simulink model "RoboBoatVU_2014_Bacchus"  (R2014a)
settings: Solver=FixedStepDiscrete  StartTime=0.0  StopTime=inf  FixedStep=.1  RelTol=1e-3
undefined symbols (not defined in the file): Com1, Com2, Com3, Com4, DiscIntNeverNeededParam, RGB24, standard
libraries: visiontextngfix x51, simulink x44, xpcseriallib x15, dspmtrx3 x14, speedgoatlib_IO102 x3, slrtlib x2, visionstatistics x2, dspstat3 x2, dspindex x2, xpcvideousblib x2, xpcvideoutillib x2, speedgoatlib x1
(part 4 of 5)

== system RoboBoatVU_2014_Bacchus/Main FSM/Start Speed Gate/Buoy Decisions/Annotate Image ==
  RGB image : Inport
  Red BBox : Inport  Port=2
  Green BBox : Inport  Port=3
  Red Dist : Inport  Port=4
  Green Dist : Inport  Port=5
  Annotate Task : visiontextngfix/Insert Text  inputType=Obsolete  theText='Buoy Navigation'  getTextLocFrom=Specify via dialog  textLoc=[10 10]  getTextColorFrom=Specify via dialog  textColor=[0 0 255]  getTextIntensityFrom=Specify via dialog  textIntensity=0  getTextOpacityFrom=Specify via dialog  textOpacity=1.0  dummyVar2=0  dummyVar3=0  dummyVar4=0  imagePorts=One multidimensional signal  isInputTransposed=off  fontFace=LucidaSansRegular  dummyVar1=0  blockFontSize=12  antiAliased=on
  Draw Green BBox : visiontextngfix/Draw Shapes  shape=Rectangles  fill=on  lineWidth=1  fillClrSource=Specify via dialog  display=User-specified value  intensity=200  color=[0 255 0]  opacity=0.6  viewport=Entire image  antialiasing=off  inType=Obsolete  imagePorts=One multidimensional signal  prodOutputMode=Binary point scaling  prodOutputWordLength=32  prodOutputFracLength=14  memoryMode=Specify word length  memoryWordLength=16  memoryFracLength=14  roundingMode=Floor  overflowMode=off
  Draw Red BBox : visiontextngfix/Draw Shapes  shape=Rectangles  fill=on  lineWidth=1  fillClrSource=Specify via dialog  display=User-specified value  intensity=200  color=[255 0 0]  opacity=0.6  viewport=Entire image  antialiasing=off  inType=Obsolete  imagePorts=One multidimensional signal  prodOutputMode=Binary point scaling  prodOutputWordLength=32  prodOutputFracLength=14  memoryMode=Specify word length  memoryWordLength=16  memoryFracLength=14  roundingMode=Floor  overflowMode=off
  Green Distance Display : visiontextngfix/Insert Text  inputType=Obsolete  theText='Green Distance: %f m'  getTextLocFrom=Specify via dialog  textLoc=[10 130]  getTextColorFrom=Specify via dialog  textColor=[0 255 0]  getTextIntensityFrom=Specify via dialog  textIntensity=0  getTextOpacityFrom=Specify via dialog  textOpacity=1.0  dummyVar2=0  dummyVar3=0  dummyVar4=0  imagePorts=One multidimensional signal  isInputTransposed=off  fontFace=LucidaSansRegular  dummyVar1=0  blockFontSize=12  antiAliased=on
  Green integer : DataTypeConversion  OutDataTypeStr=int32
  Red Distance Display : visiontextngfix/Insert Text  inputType=Obsolete  theText='Red Distance: %f m'  getTextLocFrom=Specify via dialog  textLoc=[10 70]  getTextColorFrom=Specify via dialog  textColor=[255 0 0]  getTextIntensityFrom=Specify via dialog  textIntensity=0  getTextOpacityFrom=Specify via dialog  textOpacity=1.0  dummyVar2=0  dummyVar3=0  dummyVar4=0  imagePorts=One multidimensional signal  isInputTransposed=off  fontFace=LucidaSansRegular  dummyVar1=0  blockFontSize=12  antiAliased=on
  Red integer : DataTypeConversion  OutDataTypeStr=int32
  Annotated Image : Outport
  wires:
  RGB image/1 -> Draw Red BBox/1
  Red BBox/1 -> Red integer/1
  Red integer/1 -> Draw Red BBox/2
  Draw Red BBox/1 -> Draw Green BBox/1
  Green BBox/1 -> Green integer/1
  Draw Green BBox/1 -> Annotate Task/1
  Annotate Task/1 -> Red Distance Display/1
  Red Dist/1 -> Red Distance Display/2
  Green Distance Display/1 -> Annotated Image/1
  Red Distance Display/1 -> Green Distance Display/1
  Green Dist/1 -> Green Distance Display/2
  Green integer/1 -> Draw Green BBox/2

== system RoboBoatVU_2014_Bacchus/Main FSM/Start Speed Gate/Start Speed Gate Detection/Green Detection ==
  HSV : Inport
  Blob Analysis : visionstatistics/Blob Analysis  Tag=vipblks_row_conv  area=on  centroid=on  bBox=on  majorAxis=off  minorAxis=off  angle=off  eccentricity=off  equivDiameterSq=off  extent=on  perimeter=off  maxBlobs=4  warnIfNumBlobsExceeded=on  isCount=off  useMinArea=on  minArea=130  useMaxArea=off  maxArea=6000  excludeBorderBlob=off  outDT=double  isOutVarDim=off  isFill=on  fillValues=-1  conn=8  isLabel=off  outputMode=Binary point scaling  outputWordLength=32  outputFracLength=16  firstCoeffMode=Binary point scaling  firstCoeffWordLength=16  firstCoeffFracLength=14  secondCoeffMode=Binary point scaling  secondCoeffWordLength=32  secondCoeffFracLength=16  accumMode=Binary point scaling  accumWordLength=32  accumFracLength=0  prodOutputMode=Binary point scaling  prodOutputWordLength=32  prodOutputFracLength=16  roundingMode=Floor  overflowMode=off
  Exclusions1 : Subsystem
  Image Reduction : Subsystem
  y-shift : MATLAB Function  Commented=through  TreatAsAtomicUnit=on
  Green Centroid : Outport
  Green BBox : Outport  Port=2
  wires:
  HSV/1 -> Image Reduction/1(HSV)
  Exclusions1/1(Centroid Out) -> y-shift/1(CentroidIn)
  Exclusions1/2(BBox Out) -> y-shift/2(BBoxIn)
  y-shift/1(CentroidOut) -> Green Centroid/1
  y-shift/2(BBoxOut) -> Green BBox/1
  Blob Analysis/2 -> Exclusions1/2(Centroid In)
  Blob Analysis/1 -> Exclusions1/1(Area In)
  Blob Analysis/3 -> Exclusions1/3(BBox In)
  Blob Analysis/4 -> Exclusions1/4(Extent In)
  Image Reduction/1(Green BW) -> Blob Analysis/1

== system RoboBoatVU_2014_Bacchus/Main FSM/Start Speed Gate/Start Speed Gate Detection/Red Detection ==
  HSV : Inport
  Blob Analysis : visionstatistics/Blob Analysis  Tag=vipblks_row_conv  area=on  centroid=on  bBox=on  majorAxis=off  minorAxis=off  angle=off  eccentricity=off  equivDiameterSq=off  extent=on  perimeter=off  maxBlobs=4  warnIfNumBlobsExceeded=on  isCount=off  useMinArea=on  minArea=130  useMaxArea=off  maxArea=6000  excludeBorderBlob=off  outDT=double  isOutVarDim=off  isFill=on  fillValues=-1  conn=8  isLabel=off  outputMode=Binary point scaling  outputWordLength=32  outputFracLength=16  firstCoeffMode=Binary point scaling  firstCoeffWordLength=16  firstCoeffFracLength=14  secondCoeffMode=Binary point scaling  secondCoeffWordLength=32  secondCoeffFracLength=16  accumMode=Binary point scaling  accumWordLength=32  accumFracLength=0  prodOutputMode=Binary point scaling  prodOutputWordLength=32  prodOutputFracLength=16  roundingMode=Floor  overflowMode=off
  Exclusions : Subsystem
  Image Reduction : Subsystem
  y-shift : MATLAB Function  Commented=through  TreatAsAtomicUnit=on
  Red Centroid : Outport
  Red BBox : Outport  Port=2
  wires:
  HSV/1 -> Image Reduction/1(HSV)
  Exclusions/1(Centroid Out) -> y-shift/1(CentroidIn)
  Exclusions/2(BBox Out) -> y-shift/2(BBoxIn)
  y-shift/2(BBoxOut) -> Red BBox/1
  y-shift/1(CentroidOut) -> Red Centroid/1
  Blob Analysis/4 -> Exclusions/4(Extent In)
  Blob Analysis/2 -> Exclusions/2(Centroid In)
  Blob Analysis/1 -> Exclusions/1(Area In)
  Blob Analysis/3 -> Exclusions/3(BBox In)
  Image Reduction/1(Red BW) -> Blob Analysis/1

== system RoboBoatVU_2014_Bacchus/Sensors/Serial In/Decode Compass/Correct Heading Angle Magnetic to True North ==
  Heading Mag : Inport
  Magnetic Declination : Constant  Value=-10.877
  Magnetic to True North Conversion : MATLAB Function  TreatAsAtomicUnit=on
  Heading True : Outport
  wires:
  Magnetic to True North Conversion/1(HeadingT) -> Heading True/1  "Heading"
  Heading Mag/1 -> Magnetic to True North Conversion/1(HeadingM)
  Magnetic Declination/1 -> Magnetic to True North Conversion/2(MagDec)

== system RoboBoatVU_2014_Bacchus/Sinks/actuators/analog output/Subsystem ==
  Compass Heading : Inport
  Control Signals : Inport  Port=2
  Bus Selector : BusSelector  OutputSignals=RPM,Desired Heading
  Heading Controller : Subsystem
  Propulsion Controller : Subsystem
  Propulsion : Outport
  Steering : Outport  Port=2
  wires:
  Control Signals/1 -> Bus Selector/1
  Bus Selector/1 -> Propulsion Controller/1(RPM)  "<RPM>"
  Propulsion Controller/1(Propulsion) -> Propulsion/1
  Bus Selector/2 -> Heading Controller/1(Heading Desired)  "<Desired Heading>"
  Compass Heading/1 -> Heading Controller/2(Compass Heading)
  Heading Controller/1(Steering) -> Steering/1

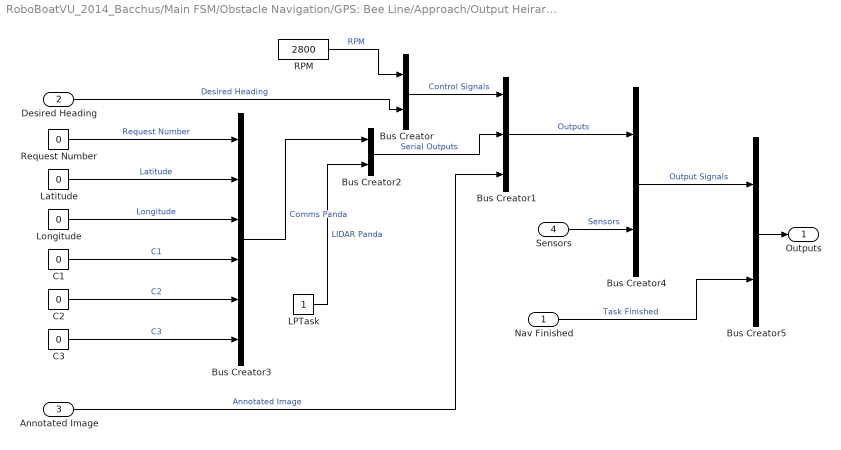
== system RoboBoatVU_2014_Bacchus/Main FSM/Obstacle Navigation/GPS: Bee Line/Approach/Output Heirarchy1 ==
  Nav Finished : Inport
  Desired Heading : Inport  Port=2
  Annotated Image : Inport  Port=3
  Sensors : Inport  Port=4
  Bus Creator{,2,4..5} (4 alike) : BusCreator  Inputs=2
  Bus Creator1 : BusCreator  Inputs=3
  Bus Creator3 : BusCreator  Inputs=6
  C1 : Constant  Value=0
  C2 : Constant  Value=0
  C3 : Constant  Value=0
  LPTask : Constant
  Latitude : Constant  Value=0
  Longitude : Constant  Value=0
  RPM : Constant  Value=2800
  Request Number : Constant  Value=0
  Outputs : Outport
  wires:
  RPM/1 -> Bus Creator/1  "RPM"
  Bus Creator/1 -> Bus Creator1/1  "Control Signals"
  Bus Creator3/1 -> Bus Creator2/1  "Comms Panda"
  Request Number/1 -> Bus Creator3/1  "Request Number"
  Latitude/1 -> Bus Creator3/2  "Latitude"
  Longitude/1 -> Bus Creator3/3  "Longitude"
  C1/1 -> Bus Creator3/4  "C1"
  LPTask/1 -> Bus Creator2/2  "LIDAR Panda"
  Desired Heading/1 -> Bus Creator/2  "Desired Heading"
  Bus Creator1/1 -> Bus Creator4/1  "Outputs"
  Annotated Image/1 -> Bus Creator1/3  "Annotated Image"
  Sensors/1 -> Bus Creator4/2  "Sensors"
  Bus Creator4/1 -> Bus Creator5/1  "Output Signals"
  Bus Creator2/1 -> Bus Creator1/2  "Serial Outputs"
  C2/1 -> Bus Creator3/5  "C2"
  C3/1 -> Bus Creator3/6  "C3"
  Nav Finished/1 -> Bus Creator5/2  "Task Finished"
  Bus Creator5/1 -> Outputs/1

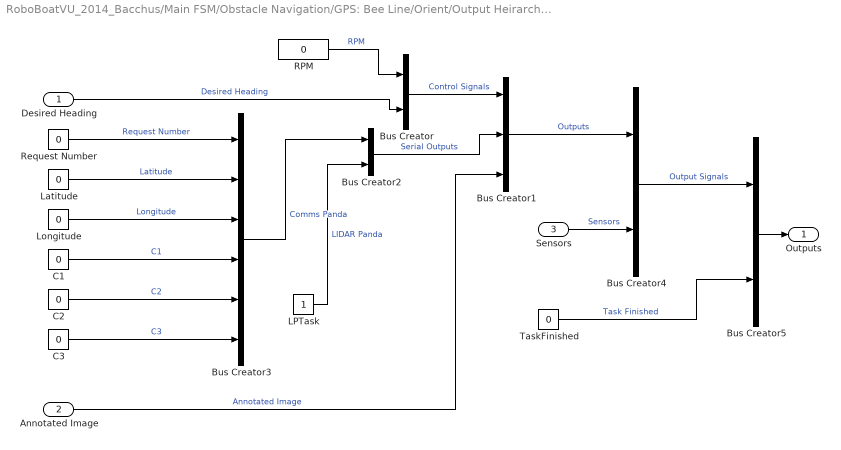
== system RoboBoatVU_2014_Bacchus/Main FSM/Obstacle Navigation/GPS: Bee Line/Orient/Output Heirarchy1 ==
  Desired Heading : Inport
  Annotated Image : Inport  Port=2
  Sensors : Inport  Port=3
  Bus Creator{,2,4..5} (4 alike) : BusCreator  Inputs=2
  Bus Creator1 : BusCreator  Inputs=3
  Bus Creator3 : BusCreator  Inputs=6
  C1 : Constant  Value=0
  C2 : Constant  Value=0
  C3 : Constant  Value=0
  LPTask : Constant
  Latitude : Constant  Value=0
  Longitude : Constant  Value=0
  RPM : Constant  Value=0
  Request Number : Constant  Value=0
  TaskFinished : Constant  Value=0
  Outputs : Outport
  wires:
  RPM/1 -> Bus Creator/1  "RPM"
  Bus Creator/1 -> Bus Creator1/1  "Control Signals"
  Bus Creator3/1 -> Bus Creator2/1  "Comms Panda"
  Request Number/1 -> Bus Creator3/1  "Request Number"
  Latitude/1 -> Bus Creator3/2  "Latitude"
  Longitude/1 -> Bus Creator3/3  "Longitude"
  C1/1 -> Bus Creator3/4  "C1"
  LPTask/1 -> Bus Creator2/2  "LIDAR Panda"
  Desired Heading/1 -> Bus Creator/2  "Desired Heading"
  Bus Creator1/1 -> Bus Creator4/1  "Outputs"
  Annotated Image/1 -> Bus Creator1/3  "Annotated Image"
  Sensors/1 -> Bus Creator4/2  "Sensors"
  Bus Creator4/1 -> Bus Creator5/1  "Output Signals"
  Bus Creator2/1 -> Bus Creator1/2  "Serial Outputs"
  C2/1 -> Bus Creator3/5  "C2"
  C3/1 -> Bus Creator3/6  "C3"
  TaskFinished/1 -> Bus Creator5/2  "Task Finished"
  Bus Creator5/1 -> Outputs/1

== system RoboBoatVU_2014_Bacchus/Main FSM/Obstacle Navigation1/Enter Gate/Gate 1 (Red & White)/Output Heirarchy ==
  Annotated Image : Inport
  Sensors : Inport  Port=2
  RPM : Inport  Port=3
  Desired Heading : Inport  Port=4
  Task Finished : Inport  Port=5
  Bus Creator : BusCreator  Inputs=3
  Bus Creator1 : BusCreator  Inputs=2
  Bus Creator2 : BusCreator  Inputs=3
  Bus Creator3 : BusCreator  Inputs=2
  Bus Creator4 : BusCreator  Inputs=2
  Due Sample Start : Constant  Value=0
  Ready to Read : Constant  Value=0
  Uno Power : Constant  Value=0
  Outputs : Outport
  wires:
  RPM/1 -> Bus Creator/1  "RPM"
  Bus Creator/1 -> Bus Creator1/1  "Control Signals"
  Bus Creator2/1 -> Bus Creator/3  "Arduino Signals"
  Uno Power/1 -> Bus Creator2/2  "Uno Power"
  Desired Heading/1 -> Bus Creator/2  "Desired Heading"
  Bus Creator1/1 -> Bus Creator4/1  "Outputs"
  Annotated Image/1 -> Bus Creator1/2  "Annotated Image"
  Sensors/1 -> Bus Creator4/2  "Sensors"
  Bus Creator4/1 -> Bus Creator3/1  "Output Signals"
  Ready to Read/1 -> Bus Creator2/1  "Ready to Read"
  Due Sample Start/1 -> Bus Creator2/3  "Due Sample Start"
  Task Finished/1 -> Bus Creator3/2  "Task Finished"
  Bus Creator3/1 -> Outputs/1

== system RoboBoatVU_2014_Bacchus/Main FSM/Obstacle Navigation1/Enter Gate/Gate 2 (White & White)/Output Heirarchy ==
  Annotated Image : Inport
  Sensors : Inport  Port=2
  RPM : Inport  Port=3
  Desired Heading : Inport  Port=4
  Task Finished : Inport  Port=5
  Bus Creator : BusCreator  Inputs=3
  Bus Creator1 : BusCreator  Inputs=2
  Bus Creator2 : BusCreator  Inputs=3
  Bus Creator3 : BusCreator  Inputs=2
  Bus Creator4 : BusCreator  Inputs=2
  Due Sample Start : Constant  Value=0
  Ready to Read : Constant  Value=0
  Uno Power : Constant  Value=0
  Outputs : Outport
  wires:
  RPM/1 -> Bus Creator/1  "RPM"
  Bus Creator/1 -> Bus Creator1/1  "Control Signals"
  Bus Creator2/1 -> Bus Creator/3  "Arduino Signals"
  Uno Power/1 -> Bus Creator2/2  "Uno Power"
  Desired Heading/1 -> Bus Creator/2  "Desired Heading"
  Bus Creator1/1 -> Bus Creator4/1  "Outputs"
  Annotated Image/1 -> Bus Creator1/2  "Annotated Image"
  Sensors/1 -> Bus Creator4/2  "Sensors"
  Bus Creator4/1 -> Bus Creator3/1  "Output Signals"
  Ready to Read/1 -> Bus Creator2/1  "Ready to Read"
  Due Sample Start/1 -> Bus Creator2/3  "Due Sample Start"
  Task Finished/1 -> Bus Creator3/2  "Task Finished"
  Bus Creator3/1 -> Outputs/1

== system RoboBoatVU_2014_Bacchus/Main FSM/Obstacle Navigation1/Enter Gate/Gate 3 (White & Green)/Output Heirarchy ==
  Annotated Image : Inport
  Sensors : Inport  Port=2
  RPM : Inport  Port=3
  Desired Heading : Inport  Port=4
  Task Finished : Inport  Port=5
  Bus Creator : BusCreator  Inputs=3
  Bus Creator1 : BusCreator  Inputs=2
  Bus Creator2 : BusCreator  Inputs=3
  Bus Creator3 : BusCreator  Inputs=2
  Bus Creator4 : BusCreator  Inputs=2
  Due Sample Start : Constant  Value=0
  Ready to Read : Constant  Value=0
  Uno Power : Constant  Value=0
  Outputs : Outport
  wires:
  RPM/1 -> Bus Creator/1  "RPM"
  Bus Creator/1 -> Bus Creator1/1  "Control Signals"
  Bus Creator2/1 -> Bus Creator/3  "Arduino Signals"
  Uno Power/1 -> Bus Creator2/2  "Uno Power"
  Desired Heading/1 -> Bus Creator/2  "Desired Heading"
  Bus Creator1/1 -> Bus Creator4/1  "Outputs"
  Annotated Image/1 -> Bus Creator1/2  "Annotated Image"
  Sensors/1 -> Bus Creator4/2  "Sensors"
  Bus Creator4/1 -> Bus Creator3/1  "Output Signals"
  Ready to Read/1 -> Bus Creator2/1  "Ready to Read"
  Due Sample Start/1 -> Bus Creator2/3  "Due Sample Start"
  Task Finished/1 -> Bus Creator3/2  "Task Finished"
  Bus Creator3/1 -> Outputs/1

== system RoboBoatVU_2014_Bacchus/Main FSM/Obstacle Navigation1/Exit Gate/Gate 1 (Red & White)/Output Heirarchy ==
  Annotated Image : Inport
  Sensors : Inport  Port=2
  RPM : Inport  Port=3
  Desired Heading : Inport  Port=4
  Task Finished : Inport  Port=5
  Bus Creator : BusCreator  Inputs=3
  Bus Creator1 : BusCreator  Inputs=2
  Bus Creator2 : BusCreator  Inputs=3
  Bus Creator3 : BusCreator  Inputs=2
  Bus Creator4 : BusCreator  Inputs=2
  Due Sample Start : Constant  Value=0
  Ready to Read : Constant  Value=0
  Uno Power : Constant  Value=0
  Outputs : Outport
  wires:
  RPM/1 -> Bus Creator/1  "RPM"
  Bus Creator/1 -> Bus Creator1/1  "Control Signals"
  Bus Creator2/1 -> Bus Creator/3  "Arduino Signals"
  Uno Power/1 -> Bus Creator2/2  "Uno Power"
  Desired Heading/1 -> Bus Creator/2  "Desired Heading"
  Bus Creator1/1 -> Bus Creator4/1  "Outputs"
  Annotated Image/1 -> Bus Creator1/2  "Annotated Image"
  Sensors/1 -> Bus Creator4/2  "Sensors"
  Bus Creator4/1 -> Bus Creator3/1  "Output Signals"
  Ready to Read/1 -> Bus Creator2/1  "Ready to Read"
  Due Sample Start/1 -> Bus Creator2/3  "Due Sample Start"
  Task Finished/1 -> Bus Creator3/2  "Task Finished"
  Bus Creator3/1 -> Outputs/1

== system RoboBoatVU_2014_Bacchus/Main FSM/Obstacle Navigation1/Exit Gate/Gate 2 (White & White)/Output Heirarchy ==
  Annotated Image : Inport
  Sensors : Inport  Port=2
  RPM : Inport  Port=3
  Desired Heading : Inport  Port=4
  Task Finished : Inport  Port=5
  Bus Creator : BusCreator  Inputs=3
  Bus Creator1 : BusCreator  Inputs=2
  Bus Creator2 : BusCreator  Inputs=3
  Bus Creator3 : BusCreator  Inputs=2
  Bus Creator4 : BusCreator  Inputs=2
  Due Sample Start : Constant  Value=0
  Ready to Read : Constant  Value=0
  Uno Power : Constant  Value=0
  Outputs : Outport
  wires:
  RPM/1 -> Bus Creator/1  "RPM"
  Bus Creator/1 -> Bus Creator1/1  "Control Signals"
  Bus Creator2/1 -> Bus Creator/3  "Arduino Signals"
  Uno Power/1 -> Bus Creator2/2  "Uno Power"
  Desired Heading/1 -> Bus Creator/2  "Desired Heading"
  Bus Creator1/1 -> Bus Creator4/1  "Outputs"
  Annotated Image/1 -> Bus Creator1/2  "Annotated Image"
  Sensors/1 -> Bus Creator4/2  "Sensors"
  Bus Creator4/1 -> Bus Creator3/1  "Output Signals"
  Ready to Read/1 -> Bus Creator2/1  "Ready to Read"
  Due Sample Start/1 -> Bus Creator2/3  "Due Sample Start"
  Task Finished/1 -> Bus Creator3/2  "Task Finished"
  Bus Creator3/1 -> Outputs/1

== system RoboBoatVU_2014_Bacchus/Main FSM/Obstacle Navigation1/Exit Gate/Gate 3 (White & Green)/Output Heirarchy ==
  Annotated Image : Inport
  Sensors : Inport  Port=2
  RPM : Inport  Port=3
  Desired Heading : Inport  Port=4
  Task Finished : Inport  Port=5
  Bus Creator : BusCreator  Inputs=3
  Bus Creator1 : BusCreator  Inputs=2
  Bus Creator2 : BusCreator  Inputs=3
  Bus Creator3 : BusCreator  Inputs=2
  Bus Creator4 : BusCreator  Inputs=2
  Due Sample Start : Constant  Value=0
  Ready to Read : Constant  Value=0
  Uno Power : Constant  Value=0
  Outputs : Outport
  wires:
  RPM/1 -> Bus Creator/1  "RPM"
  Bus Creator/1 -> Bus Creator1/1  "Control Signals"
  Bus Creator2/1 -> Bus Creator/3  "Arduino Signals"
  Uno Power/1 -> Bus Creator2/2  "Uno Power"
  Desired Heading/1 -> Bus Creator/2  "Desired Heading"
  Bus Creator1/1 -> Bus Creator4/1  "Outputs"
  Annotated Image/1 -> Bus Creator1/2  "Annotated Image"
  Sensors/1 -> Bus Creator4/2  "Sensors"
  Bus Creator4/1 -> Bus Creator3/1  "Output Signals"
  Ready to Read/1 -> Bus Creator2/1  "Ready to Read"
  Due Sample Start/1 -> Bus Creator2/3  "Due Sample Start"
  Task Finished/1 -> Bus Creator3/2  "Task Finished"
  Bus Creator3/1 -> Outputs/1

== system RoboBoatVU_2014_Bacchus/Main FSM/Obstacle Navigation1/GPS: Center/Approach/Output Heirarchy ==
  Finished : Inport
  Desired Heading : Inport  Port=2
  Annotated Image : Inport  Port=3
  Sensors : Inport  Port=4
  Bus Creator : BusCreator  Inputs=3
  Bus Creator1 : BusCreator  Inputs=2
  Bus Creator2 : BusCreator  Inputs=3
  Bus Creator3 : BusCreator  Inputs=2
  Bus Creator4 : BusCreator  Inputs=2
  Due Sample Start : Constant  Value=0
  RPM Desired : Constant  Value=4000
  Ready to Read : Constant  Value=0
  Uno Power : Constant  Value=0
  Outputs : Outport
  wires:
  RPM Desired/1 -> Bus Creator/1  "RPM"
  Bus Creator/1 -> Bus Creator1/1  "Control Signals"
  Bus Creator2/1 -> Bus Creator/3  "Arduino Signals"
  Uno Power/1 -> Bus Creator2/2  "Uno Power"
  Desired Heading/1 -> Bus Creator/2  "Desired Heading"
  Bus Creator1/1 -> Bus Creator4/1  "Outputs"
  Annotated Image/1 -> Bus Creator1/2  "Annotated Image"
  Sensors/1 -> Bus Creator4/2  "Sensors"
  Bus Creator4/1 -> Bus Creator3/1  "Output Signals"
  Ready to Read/1 -> Bus Creator2/1  "Ready to Read"
  Due Sample Start/1 -> Bus Creator2/3  "Due Sample Start"
  Bus Creator3/1 -> Outputs/1
  Finished/1 -> Bus Creator3/2  "Task Finished"

== matlab function RoboBoatVU_2014_Bacchus/Main FSM/Obstacle Navigation/GPS: Bee Line/Orient/Desired Heading ==
  data: DesiredGPS input; DesiredHeading output; GPSLat input; GPSLong input
function DesiredHeading = Orient(DesiredGPS, GPSLat, GPSLong)

%Written by Anderson Lebbad on July 22, 2013
%Last Edited: Edward Zhu on July 5, 2014

% Edit:
% Changed calculation to use positive lat and negative long

%Orients the boat towards a target GPS point before approaching it.
%This is done to keep the approach angle minimal, so the approach
%algorithm does not circle the target and never reach it.

%Parse input GPS and convert angles to radians
CurLat = (floor(GPSLat/100)+mod(GPSLat,100)/60)*pi/180;
CurLong = (ceil(GPSLong/100)-mod(-GPSLong,100)/60)*pi/180;
DesLat = (floor(DesiredGPS(1)/100)+mod(DesiredGPS(1),100)/60)*pi/180;
DesLong = (ceil(DesiredGPS(2)/100)-mod(-DesiredGPS(2),100)/60)*pi/180;

%Difference between longs
DiffLong = DesLong - CurLong;

%Calculate initial bearing - formula documented here: 
%   http://www.movable-type.co.uk/scripts/latlong.html
y = sin(DiffLong)*cos(DesLat);
x = cos(CurLat)*sin(DesLat)-sin(CurLat)*cos(DesLat)*cos(DiffLong);
DesiredHeading = mod(atan2(y, x)*180/pi + 360, 360);

== matlab function RoboBoatVU_2014_Bacchus/Main FSM/Obstacle Navigation1/Enter Gate/Gate 2 (White & White)/Distance ==
  data: Distance output; DesiredGPS input; GPSLat input; GPSLong input
function Distance  = DistCalc(DesiredGPS, GPSLat, GPSLong)

%Written by Anderson Lebbad on July 22, 2013
%Last Edited:

%Orients the boat towards a target GPS point before approaching it.
%This is done to keep the approach angle minimal, so the approach
%algorithm does not circle the target and never reach it.

%Parse input GPS and convert angles to radians
CurLat = (floor(GPSLat/100)+mod(GPSLat,100)/60)*pi/180;
CurLong = (floor(GPSLong/100)+mod(GPSLong,100)/60)*pi/180;
DesLat = (floor(DesiredGPS(1)/100)+mod(DesiredGPS(1),100)/60)*pi/180;
DesLong = (floor(DesiredGPS(2)/100)+mod(DesiredGPS(2),100)/60)*pi/180;
%Difference between lats and longs
DiffLat = DesLat - CurLat;
MidLat = cos((CurLat + DesLat)/2);
DiffLong = DesLong - CurLong;
%Radius of the earth in meters
R = 6378137;

%Calculate distance using the great-circle distance formula
%Formula documented here:
%   http://www.movable-type.co.uk/scripts/latlong.html
% a = sin(DiffLat/2)^2+sin(DiffLong/2)^2*cos(CurLat)*cos(DesLat);
% c = 2*atan2(sqrt(a), sqrt(1-a));
% Distance = R*c;

%Calculating distance using Pythagora's
a = DiffLong*MidLat;
b = DiffLat;
Distance = R*sqrt(a^2+b^2);

== matlab function RoboBoatVU_2014_Bacchus/Main FSM/Obstacle Navigation1/Enter Gate/Gate 3 (White & Green)/MATLAB Function ==
  data: Prob input; RPM output; ColorID input; Dist input; Ang input; CurrentHeading input; GPSLat input; GPSLong input; Timer input; DesiredHeading output; gateGPS output
function [RPM,DesiredHeading,gateGPS] = navigation(Prob,ColorID,Dist,Ang,CurrentHeading,GPSLat,GPSLong,Timer)

% Function performs one buoy navigation through the start speed gates. If
% no buoys are found by the LIDAR/Vision assembly then an incremented
% turning algorithm is executed to turn by 10 degrees per increment up to 
% 90 degrees either way of the inital heading

% Written by Edward Zhu


persistent LockHeading TimeLastFound Counter Turn TurnInc gateLat gateLong

if isempty(LockHeading) && isempty(TimeLastFound) && isempty(Counter) && isempty(Turn) && isempty(TurnInc)
    LockHeading = CurrentHeading;
    TimeLastFound = 0;
    Counter = 0;
    TurnInc = 30;
    Turn = TurnInc;
    gateLat = 0;
    gateLong = 0;
end
Distance = Dist/100;
BoatWidth = 0.75;
Buffer = atan(2*BoatWidth/Distance);

WhiteOffset = Ang + Buffer;
GreenOffset = Ang - Buffer;

R = 6378137;

CurLat = (floor(GPSLat/100)+mod(GPSLat,100)/60)*pi/180;
CurLong = (ceil(GPSLong/100)-mod(-GPSLong,100)/60)*pi/180;

gateHeading = (mod(CurrentHeading - Ang, 360))*pi/180;

if ColorID == 2 && Prob > 0.9
    DesiredHeading = mod(LockHeading - Turn, 360);
    RPM = 0;
    GateFound = 1;
    TimeLastFound = Timer;
elseif ColorID == 3 && Prob > 0.9
    if Ang > 0
        DesiredHeading = mod(CurrentHeading - GreenOffset, 360);
    else
        DesiredHeading = mod(CurrentHeading + GreenOffset, 360);
    end
    RPM = 4000;
    GateFound = 1;
    TimeLastFound = Timer;
    gateLat =  asin(sin(CurLat)*cos(Distance/R) + cos(CurLat)*sin(Distance/R)*cos(gateHeading))*180/pi;
    gateLong = (CurLong + atan2(sin(gateHeading)*sin(Distance/R)*cos(CurLat),cos(Distance/R)-sin(CurLat)*sin(gateLat)))*180/pi;
else
    DesiredHeading = CurrentHeading;
    RPM = 0;
    GateFound = 0;
end

gateGPS = [gateLat gateLong];
TimeNoBuoys = Timer - TimeLastFound;

if GateFound == 0 && TimeNoBuoys > 15
    RPM = 0;
    DesiredHeading = mod(LockHeading - Turn, 360);
    HeadingDiff = DesiredHeading - CurrentHeading;
    gateGPS = [gateLat gateLong];
    
    if HeadingDiff > 180
        HeadingDiff = HeadingDiff - 360;
    elseif HeadingDiff < -180
        HeadingDiff = HeadingDiff + 360;
    end
    
    if HeadingDiff < 3
        Counter = Counter + 1;
    else
        Counter = 0;
    end
    
    if Counter >= 15
        Turn = Turn + TurnInc;
        Counter = 0;
        if abs(Turn) > 90
            TurnInc = -TurnInc;
        end
    end
end

== matlab function RoboBoatVU_2014_Bacchus/Main FSM/Obstacle Navigation1/GPS: Center/Orient/Desired Heading ==
  data: DesiredGPS input; DesiredHeading output; GPSLat input; GPSLong input
function DesiredHeading = Orient(DesiredGPS, GPSLat, GPSLong)

%Written by Anderson Lebbad on July 22, 2013
%Last Edited: Edward Zhu on July 5, 2014

% Edit:
% Changed calculation to use positive lat and negative long

%Orients the boat towards a target GPS point before approaching it.
%This is done to keep the approach angle minimal, so the approach
%algorithm does not circle the target and never reach it.

%Parse input GPS and convert angles to radians
CurLat = (floor(GPSLat/100)+mod(GPSLat,100)/60)*pi/180;
CurLong = (ceil(GPSLong/100)-mod(-GPSLong,100)/60)*pi/180;
DesLat = (floor(DesiredGPS(1)/100)+mod(DesiredGPS(1),100)/60)*pi/180;
DesLong = (ceil(DesiredGPS(2)/100)-mod(-DesiredGPS(2),100)/60)*pi/180;

%Difference between longs
DiffLong = DesLong - CurLong;

%Calculate initial bearing - formula documented here: 
%   http://www.movable-type.co.uk/scripts/latlong.html
y = sin(DiffLong)*cos(DesLat);
x = cos(CurLat)*sin(DesLat)-sin(CurLat)*cos(DesLat)*cos(DiffLong);
DesiredHeading = mod(atan2(y, x)*180/pi + 360, 360);

== matlab function RoboBoatVU_2014_Bacchus/Main FSM/Obstacle Navigation1/Obstacle Navigation/GPS: Bee Line/Approach/Desired Heading and Distance ==
  data: Distance output; DesiredGPS input; DesiredHeading output; GPSLat input; GPSLong input
function [Distance, DesiredHeading] = Approach(DesiredGPS, GPSLat, GPSLong)

%Written by Anderson Lebbad on July 22, 2013
%Last Edited: Edward Zhu July 5, 2014

%Edit:
% Switched from great-circle distance formula to equirectangular approx and
%used mod for desired heading
% Changed calculation to use positve lat and negative long

%Orients the boat towards a target GPS point before approaching it.
%This is done to keep the approach angle minimal, so the approach
%algorithm does not circle the target and never reach it.

%Parse input GPS and convert angles to radians
CurLat = (floor(GPSLat/100)+mod(GPSLat,100)/60)*pi/180;
CurLong = (ceil(GPSLong/100)-mod(-GPSLong,100)/60)*pi/180;
DesLat = (floor(DesiredGPS(1)/100)+mod(DesiredGPS(1),100)/60)*pi/180;
DesLong = (ceil(DesiredGPS(2)/100)-mod(-DesiredGPS(2),100)/60)*pi/180;

%Difference between lats and longs
DiffLat = DesLat - CurLat;
MidLat = cos((CurLat + DesLat)/2);
DiffLong = DesLong - CurLong;

%Radius of the earth in meters
R = 6378137;

%Calculate distance using the great-circle distance formula
%Formula documented here:
%   http://www.movable-type.co.uk/scripts/latlong.html
% a = sin(DiffLat/2)^2+sin(DiffLong/2)^2*cos(CurLat)*cos(DesLat);
% c = 2*atan2(sqrt(a), sqrt(1-a));
% Distance = R*c;

%Calculating distance using equirectangular approximation since distances
%concerned are very small
a = DiffLong*MidLat;
b = DiffLat;
Distance = R*sqrt(a^2+b^2);

%Calculate initial bearing - formula documented here: 
%   http://www.movable-type.co.uk/scripts/latlong.html
y = sin(DiffLong)*cos(DesLat);
x = cos(CurLat)*sin(DesLat)-sin(CurLat)*cos(DesLat)*cos(DiffLong);
DesiredHeading = mod(atan2(y, x)*180/pi + 360, 360);

== matlab function RoboBoatVU_2014_Bacchus/Main FSM/Start Speed Gate/Nav Finished ==
  data: Timer input; Finished output; Timeout input; DesiredGPS input; GPSLat input; GPSLong input
function Finished = NavFinished(Timer, Timeout, DesiredGPS, GPSLat, GPSLong)

%Written by Anderson Lebbad on August 23, 2013
%Last Edited by:

%Checks the timeout and GPS location to determine if the navigation block
%is done. If either one is flagged, the finished signal is sent.


%Parse input GPS and convert angles to radians
CurLat = (floor(GPSLat/100)+mod(GPSLat,100)/60)*pi/180;
CurLong = (ceil(GPSLong/100)-mod(-GPSLong,100)/60)*pi/180;
DesLat = (floor(DesiredGPS(1)/100)+mod(DesiredGPS(1),100)/60)*pi/180;
DesLong = (ceil(DesiredGPS(2)/100)-mod(-DesiredGPS(2),100)/60)*pi/180;

%Difference between lats and longs
DiffLat = DesLat - CurLat;
MidLat = cos((CurLat + DesLat)/2);
DiffLong = DesLong - CurLong;

%Radius of the earth in meters
R = 6378137;

%Calculate distance using the great-circle distance formula
%Formula documented here:
%   http://www.movable-type.co.uk/scripts/latlong.html
% a = sin(DiffLat/2)^2+sin(DiffLong/2)^2*cos(CurLat)*cos(DesLat);
% c = 2*atan2(sqrt(a), sqrt(1-a));
% Distance = R*c;

%Calculating distance using equirectangular approximation since distances
%concerned are very small
a = DiffLong*MidLat;
b = DiffLat;
Distance = R*sqrt(a^2+b^2);

%Initialize output
Finished = 0;

%Check timeout and distance, minimum distance to pass a finished signal is
%set to 2 meters
if (Timer > Timeout) || (Distance < 10)
    Finished = 1;
end

== system RoboBoatVU_2014_Bacchus/Main FSM/Obstacle Navigation1/GPS: Center/Orient/Output Heirarchy1 ==
  Annotated Image : Inport
  Desired Heading : Inport  Port=2
  Sensors : Inport  Port=3
  Bus Creator : BusCreator  Inputs=3
  Bus Creator1 : BusCreator  Inputs=2
  Bus Creator2 : BusCreator  Inputs=3
  Bus Creator3 : BusCreator  Inputs=2
  Bus Creator4 : BusCreator  Inputs=2
  Due Sample Start : Constant  Value=0
  Finished : Constant  Value=0
  RPM Desired : Constant  Value=0
  Ready to Read : Constant  Value=0
  Uno Power : Constant  Value=0
  Outputs : Outport
  wires:
  RPM Desired/1 -> Bus Creator/1  "RPM"
  Bus Creator/1 -> Bus Creator1/1  "Control Signals"
  Bus Creator2/1 -> Bus Creator/3  "Arduino Signals"
  Uno Power/1 -> Bus Creator2/2  "Uno Power"
  Desired Heading/1 -> Bus Creator/2  "Desired Heading"
  Bus Creator1/1 -> Bus Creator4/1  "Outputs"
  Annotated Image/1 -> Bus Creator1/2  "Annotated Image"
  Sensors/1 -> Bus Creator4/2  "Sensors"
  Bus Creator4/1 -> Bus Creator3/1  "Output Signals"
  Ready to Read/1 -> Bus Creator2/1  "Ready to Read"
  Due Sample Start/1 -> Bus Creator2/3  "Due Sample Start"
  Bus Creator3/1 -> Outputs/1
  Finished/1 -> Bus Creator3/2  "Task Finished"

== system RoboBoatVU_2014_Bacchus/Main FSM/Obstacle Navigation1/Obstacle Navigation/Dodge/Output Heirarchy ==
  Annotated Image : Inport
  Sensors : Inport  Port=2
  RPM : Inport  Port=3
  Desired Heading : Inport  Port=4
  Bus Creator : BusCreator  Inputs=3
  Bus Creator1 : BusCreator  Inputs=2
  Bus Creator2 : BusCreator  Inputs=3
  Bus Creator3 : BusCreator  Inputs=2
  Bus Creator4 : BusCreator  Inputs=2
  Due Sample Start : Constant  Value=0
  Nav Finished : Constant  Value=0
  Ready to Read : Constant  Value=0
  Uno Power : Constant  Value=0
  Outputs : Outport
  wires:
  RPM/1 -> Bus Creator/1  "RPM"
  Bus Creator/1 -> Bus Creator1/1  "Control Signals"
  Bus Creator2/1 -> Bus Creator/3  "Arduino Signals"
  Uno Power/1 -> Bus Creator2/2  "Uno Power"
  Desired Heading/1 -> Bus Creator/2  "Desired Heading"
  Bus Creator1/1 -> Bus Creator4/1  "Outputs"
  Annotated Image/1 -> Bus Creator1/2  "Annotated Image"
  Sensors/1 -> Bus Creator4/2  "Sensors"
  Bus Creator4/1 -> Bus Creator3/1  "Output Signals"
  Ready to Read/1 -> Bus Creator2/1  "Ready to Read"
  Due Sample Start/1 -> Bus Creator2/3  "Due Sample Start"
  Bus Creator3/1 -> Outputs/1
  Nav Finished/1 -> Bus Creator3/2  "Task Finished"

== system RoboBoatVU_2014_Bacchus/Main FSM/Obstacle Navigation1/Obstacle Navigation/GPS: Bee Line/Approach ==
  Sensors : Inport
  RGB image : Inport  Port=2
  Enable : EnablePort
  Annotate Task : visiontextngfix/Insert Text  inputType=Obsolete  theText='GPS - Start: Approach - Distance: %f'  getTextLocFrom=Specify via dialog  textLoc=[10 70]  getTextColorFrom=Specify via dialog  textColor=[255 0 0]  getTextIntensityFrom=Specify via dialog  textIntensity=0  getTextOpacityFrom=Specify via dialog  textOpacity=1.0  dummyVar2=0  dummyVar3=0  dummyVar4=0  imagePorts=One multidimensional signal  isInputTransposed=off  fontFace=LucidaSansRegular  dummyVar1=0  blockFontSize=12  antiAliased=on
  Annotate Task2 : visiontextngfix/Insert Text  inputType=Obsolete  theText='Bee Line Approach'  getTextLocFrom=Specify via dialog  textLoc=[1 1]  getTextColorFrom=Specify via dialog  textColor=[0 0 0]  getTextIntensityFrom=Specify via dialog  textIntensity=0  getTextOpacityFrom=Specify via dialog  textOpacity=1.0  dummyVar2=0  dummyVar3=0  dummyVar4=0  imagePorts=One multidimensional signal  isInputTransposed=off  fontFace=LucidaSansRegular  dummyVar1=0  blockFontSize=12  antiAliased=on
  Annotate Task3 : visiontextngfix/Insert Text  inputType=Obsolete  theText='Obstacle- Distance: %f'  getTextLocFrom=Specify via dialog  textLoc=[10 100]  getTextColorFrom=Specify via dialog  textColor=[255 0 0]  getTextIntensityFrom=Specify via dialog  textIntensity=0  getTextOpacityFrom=Specify via dialog  textOpacity=1.0  dummyVar2=0  dummyVar3=0  dummyVar4=0  imagePorts=One multidimensional signal  isInputTransposed=off  fontFace=LucidaSansRegular  dummyVar1=0  blockFontSize=12  antiAliased=on
  Bus Selector : BusSelector  OutputSignals=Serial In.GPS.latitude,Serial In.GPS.longitude,Serial In.Buoy Info.Color ID,Serial In.Buoy Info.Distance
  Compare To Constant : simulink/Logic and Bit Operations/Compare To Constant  relop=<=  const=5  OutDataTypeStr=boolean
  Data Store Read : DataStoreRead  DataStoreName=obstNavEndGPS  SampleTime=0.1
  Data Type Conversion : DataTypeConversion  OutDataTypeStr=double
  Desired Heading and Distance : MATLAB Function  TreatAsAtomicUnit=on
  Obstacle Distance : MATLAB Function  TreatAsAtomicUnit=on
  Output Heirarchy : Subsystem
  Outputs : Outport
  Dodge Start : Outport  Port=2
  wires:
  Sensors/1 -> Output Heirarchy/3(Sensors), Bus Selector/1  "Sensors"
  Data Store Read/1 -> Desired Heading and Distance/1(DesiredGPS)
  Bus Selector/1 -> Desired Heading and Distance/2(GPSLat)  "<latitude>"
  Bus Selector/2 -> Desired Heading and Distance/3(GPSLong)  "<longitude>"
  Desired Heading and Distance/2(DesiredHeading) -> Output Heirarchy/2(Desired Heading)
  RGB image/1 -> Annotate Task2/1
  Desired Heading and Distance/1(Distance) -> Compare To Constant/1, Annotate Task/2
  Data Type Conversion/1 -> Output Heirarchy/1(Nav Finished)  "Task Finished"
  Output Heirarchy/1(Outputs) -> Outputs/1
  Annotate Task2/1 -> Annotate Task/1
  Annotate Task/1 -> Annotate Task3/1
  Annotate Task3/1 -> Output Heirarchy/4(Annotated Image)
  Obstacle Distance/2(DodgeStart) -> Dodge Start/1
  Compare To Constant/1 -> Data Type Conversion/1
  Obstacle Distance/1(ObstDist) -> Annotate Task3/2
  Bus Selector/3 -> Obstacle Distance/1(ColorID)  "<Color ID>"
  Bus Selector/4 -> Obstacle Distance/2(Dist)  "<Distance>"

== system RoboBoatVU_2014_Bacchus/Main FSM/Obstacle Navigation1/Obstacle Navigation/GPS: Bee Line/Orient ==
  Sensors : Inport
  RGB image : Inport  Port=2
  Enable : EnablePort
  Annotate Task : visiontextngfix/Insert Text  inputType=Obsolete  theText='GPS - Center: Orient %f'  getTextLocFrom=Specify via dialog  textLoc=[10 70]  getTextColorFrom=Specify via dialog  textColor=[255 0 0]  getTextIntensityFrom=Specify via dialog  textIntensity=0  getTextOpacityFrom=Specify via dialog  textOpacity=1.0  dummyVar2=0  dummyVar3=0  dummyVar4=0  imagePorts=One multidimensional signal  isInputTransposed=off  fontFace=LucidaSansRegular  dummyVar1=0  blockFontSize=12  antiAliased=on
  Annotate Task1 : visiontextngfix/Insert Text  inputType=Obsolete  theText='Current Heading %f'  getTextLocFrom=Specify via dialog  textLoc=[10 40]  getTextColorFrom=Specify via dialog  textColor=[255 0 0]  getTextIntensityFrom=Specify via dialog  textIntensity=0  getTextOpacityFrom=Specify via dialog  textOpacity=1.0  dummyVar2=0  dummyVar3=0  dummyVar4=0  imagePorts=One multidimensional signal  isInputTransposed=off  fontFace=LucidaSansRegular  dummyVar1=0  blockFontSize=12  antiAliased=on
  Annotate Task2 : visiontextngfix/Insert Text  inputType=Obsolete  theText='Bee Line Orient'  getTextLocFrom=Specify via dialog  textLoc=[1 1]  getTextColorFrom=Specify via dialog  textColor=[0 0 0]  getTextIntensityFrom=Specify via dialog  textIntensity=0  getTextOpacityFrom=Specify via dialog  textOpacity=1.0  dummyVar2=0  dummyVar3=0  dummyVar4=0  imagePorts=One multidimensional signal  isInputTransposed=off  fontFace=LucidaSansRegular  dummyVar1=0  blockFontSize=12  antiAliased=on
  Bus Selector : BusSelector  OutputSignals=Serial In.GPS.latitude,Serial In.GPS.longitude,Serial In.Compass.Heading
  Data Store Read1 : DataStoreRead  DataStoreName=obstNavEndGPS  SampleTime=0.1
  Desired Heading : MATLAB Function  TreatAsAtomicUnit=on
  Output Heirarchy1 : Subsystem
  Within Range : MATLAB Function  TreatAsAtomicUnit=on
  Outputs : Outport
  Finished : Outport  Port=2
  wires:
  Sensors/1 -> Output Heirarchy1/3(Sensors), Bus Selector/1  "Sensors"
  Data Store Read1/1 -> Desired Heading/1(DesiredGPS)
  Bus Selector/1 -> Desired Heading/2(GPSLat)  "<latitude>"
  Bus Selector/2 -> Desired Heading/3(GPSLong)  "<longitude>"
  Desired Heading/1(DesiredHeading) -> Output Heirarchy1/2(Desired Heading), Annotate Task/2, Within Range/1(DesiredHeading)
  Bus Selector/3 -> Annotate Task1/2, Within Range/2(Compass)  "<Heading>"
  Within Range/1(Finished) -> Finished/1
  RGB image/1 -> Annotate Task2/1
  Output Heirarchy1/1(Outputs) -> Outputs/1
  Annotate Task/1 -> Annotate Task1/1
  Annotate Task1/1 -> Output Heirarchy1/1(Annotated Image)
  Annotate Task2/1 -> Annotate Task/1

== system RoboBoatVU_2014_Bacchus/Main FSM/Start Speed Gate/Start Speed Gate Detection/Green Detection/Exclusions1 ==
  Area In : Inport
  Centroid In : Inport  Port=2
  BBox In : Inport  Port=3
  Extent In : Inport  Port=4
  Closest Blob : Subsystem
  Data Type Conversion : DataTypeConversion  OutDataTypeStr=double
  Extent Exclusion : Subsystem
  Height to Width Exclusion : Subsystem
  Logical Operator : Logic  AllPortsSameDT=off  OutDataTypeStr=boolean
  Variable Selector : dspindex/Variable Selector  NumInputs=3  rowsOrCols=Rows  IdxMode=Variable  Elements=[1 3]  ZerOneIdxMode=One-based  errmode=Clip Index  FillMode=on  FillValues=-1
  Centroid Out : Outport
  BBox Out : Outport  Port=2
  wires:
  Extent In/1 -> Extent Exclusion/1(Extent)
  BBox In/1 -> Data Type Conversion/1
  Height to Width Exclusion/1(Idx) -> Logical Operator/1
  Extent Exclusion/1(Idx) -> Logical Operator/2
  Centroid In/1 -> Variable Selector/2
  Closest Blob/1(Centroid Out) -> Centroid Out/1
  Closest Blob/2(BBox Out) -> BBox Out/1
  Data Type Conversion/1 -> Variable Selector/3, Height to Width Exclusion/1(BBox)
  Logical Operator/1 -> Variable Selector/4
  Variable Selector/3 -> Closest Blob/3(BBox In)
  Variable Selector/2 -> Closest Blob/2(Centroid In)
  Variable Selector/1 -> Closest Blob/1(Area In)
  Area In/1 -> Variable Selector/1

== system RoboBoatVU_2014_Bacchus/Main FSM/Start Speed Gate/Start Speed Gate Detection/Green Detection/Image Reduction ==
  HSV : Inport
  Cut Out Sky : dspmtrx3/Submatrix  RowSpan=Range of rows  RowStartMode=First  RowStartIndex=1  RowEndMode=Index  RowEndIndex=280  ColSpan=Range of columns  ColStartMode=First  ColStartIndex=1  ColEndMode=Last  ColEndIndex=1
  Cut Out Sky1 : dspmtrx3/Submatrix  RowSpan=Range of rows  RowStartMode=First  RowStartIndex=1  RowEndMode=Index  RowEndIndex=280  ColSpan=Range of columns  ColStartMode=First  ColStartIndex=1  ColEndMode=Last  ColEndIndex=1
  H : Selector  NumberOfDimensions=3  InputPortWidth=3  IndexOptions=Select all,Select all,Index vector (dialog)  Indices=[1 3],1,1  OutputSizes=1,1,1
  Logical Operator : Logic  AllPortsSameDT=off  OutDataTypeStr=boolean
  Logical Operator1 : Logic  AllPortsSameDT=off  OutDataTypeStr=boolean
  Logical Operator2 : Logic  AllPortsSameDT=off  OutDataTypeStr=boolean
  Upper limit : simulink/Logic and Bit Operations/Compare To Constant  relop=<=  const=110  OutDataTypeStr=boolean
  Upper limit1 : simulink/Logic and Bit Operations/Compare To Constant  relop=>=  const=90  OutDataTypeStr=boolean
  Upper limit2 : simulink/Logic and Bit Operations/Compare To Constant  relop=>=  const=60  OutDataTypeStr=boolean
  Upper limit3 : simulink/Logic and Bit Operations/Compare To Constant  relop=<=  const=160  OutDataTypeStr=boolean
  V : Selector  NumberOfDimensions=3  InputPortWidth=3  IndexOptions=Select all,Select all,Index vector (dialog)  Indices=[1 3],1,3  OutputSizes=1,1,1
  Green BW : Outport
  wires:
  H/1 -> Cut Out Sky/1
  HSV/1 -> V/1, H/1
  Cut Out Sky/1 -> Upper limit1/1, Upper limit/1
  Upper limit1/1 -> Logical Operator/2
  Upper limit/1 -> Logical Operator/1
  V/1 -> Cut Out Sky1/1
  Cut Out Sky1/1 -> Upper limit3/1, Upper limit2/1
  Logical Operator/1 -> Logical Operator1/1
  Logical Operator1/1 -> Green BW/1
  Upper limit2/1 -> Logical Operator2/1
  Upper limit3/1 -> Logical Operator2/2
  Logical Operator2/1 -> Logical Operator1/2

== system RoboBoatVU_2014_Bacchus/Main FSM/Start Speed Gate/Start Speed Gate Detection/Red Detection/Exclusions ==
  Area In : Inport
  Centroid In : Inport  Port=2
  BBox In : Inport  Port=3
  Extent In : Inport  Port=4
  Closest Blob : Subsystem
  Data Type Conversion : DataTypeConversion  OutDataTypeStr=double
  Extent Exclusion : Subsystem
  Height to Width Exclusion : Subsystem
  Logical Operator : Logic  AllPortsSameDT=off  OutDataTypeStr=boolean
  Variable Selector : dspindex/Variable Selector  NumInputs=3  rowsOrCols=Rows  IdxMode=Variable  Elements=[1 3]  ZerOneIdxMode=One-based  errmode=Clip Index  FillMode=on  FillValues=-1
  Centroid Out : Outport
  BBox Out : Outport  Port=2
  wires:
  Extent In/1 -> Extent Exclusion/1(Extent)
  BBox In/1 -> Data Type Conversion/1
  Height to Width Exclusion/1(Idx) -> Logical Operator/1
  Extent Exclusion/1(Idx) -> Logical Operator/2
  Logical Operator/1 -> Variable Selector/4
  Centroid In/1 -> Variable Selector/2
  Variable Selector/2 -> Closest Blob/2(Centroid In)
  Variable Selector/3 -> Closest Blob/3(BBox In)
  Closest Blob/1(Centroid Out) -> Centroid Out/1
  Closest Blob/2(BBox Out) -> BBox Out/1
  Data Type Conversion/1 -> Variable Selector/3, Height to Width Exclusion/1(BBox)
  Area In/1 -> Variable Selector/1
  Variable Selector/1 -> Closest Blob/1(Area In)

== system RoboBoatVU_2014_Bacchus/Main FSM/Start Speed Gate/Start Speed Gate Detection/Red Detection/Image Reduction ==
  HSV : Inport
  Cut Out Sky : dspmtrx3/Submatrix  RowSpan=Range of rows  RowStartMode=First  RowStartIndex=1  RowEndMode=Index  RowEndIndex=280  ColSpan=Range of columns  ColStartMode=First  ColStartIndex=1  ColEndMode=Last  ColEndIndex=1
  Cut Out Sky1 : dspmtrx3/Submatrix  RowSpan=Range of rows  RowStartMode=First  RowStartIndex=1  RowEndMode=Index  RowEndIndex=280  ColSpan=Range of columns  ColStartMode=First  ColStartIndex=1  ColEndMode=Last  ColEndIndex=1
  H : Selector  NumberOfDimensions=3  InputPortWidth=3  IndexOptions=Select all,Select all,Index vector (dialog)  Indices=[1 3],1,1  OutputSizes=1,1,1
  H Range 1 : simulink/Logic and Bit Operations/Compare To Constant  relop=<=  const=5  OutDataTypeStr=boolean
  H Range 2 : simulink/Logic and Bit Operations/Compare To Constant  relop=>=  const=0  OutDataTypeStr=boolean
  H Range 3 : simulink/Logic and Bit Operations/Compare To Constant  relop=<=  const=255  OutDataTypeStr=boolean
  H Range 4 : simulink/Logic and Bit Operations/Compare To Constant  relop=>=  const=220  OutDataTypeStr=boolean
  Logical Operator{,1,3..4} (4 alike) : Logic  AllPortsSameDT=off  OutDataTypeStr=boolean
  Logical Operator2 : Logic  Operator=OR  AllPortsSameDT=off  OutDataTypeStr=boolean
  V : Selector  NumberOfDimensions=3  InputPortWidth=3  IndexOptions=Select all,Select all,Index vector (dialog)  Indices=[1 3],1,3  OutputSizes=1,1,1
  V Range : simulink/Logic and Bit Operations/Compare To Constant  relop=>=  const=60  OutDataTypeStr=boolean
  V Range1 : simulink/Logic and Bit Operations/Compare To Constant  relop=<=  const=200  OutDataTypeStr=boolean
  Red BW : Outport
  wires:
  HSV/1 -> H/1, V/1
  H/1 -> Cut Out Sky/1
  Cut Out Sky/1 -> H Range 4/1, H Range 3/1, H Range 2/1, H Range 1/1
  V/1 -> Cut Out Sky1/1
  H Range 1/1 -> Logical Operator/1
  H Range 2/1 -> Logical Operator/2
  H Range 3/1 -> Logical Operator1/1
  H Range 4/1 -> Logical Operator1/2
  Logical Operator/1 -> Logical Operator2/1
  Logical Operator1/1 -> Logical Operator2/2
  Cut Out Sky1/1 -> V Range1/1, V Range/1
  Logical Operator2/1 -> Logical Operator3/1
  Logical Operator3/1 -> Red BW/1
  V Range/1 -> Logical Operator4/1
  V Range1/1 -> Logical Operator4/2
  Logical Operator4/1 -> Logical Operator3/2

== system RoboBoatVU_2014_Bacchus/Sinks/actuators/analog output/Subsystem/Heading Controller ==
  Heading Desired : Inport
  Compass Heading : Inport  Port=2
  Gain : Gain  Gain=-0.05
  MATLAB Function : MATLAB Function  TreatAsAtomicUnit=on
  Saturation : Saturate  UpperLimit=5  LowerLimit=0
  Sum : Sum  Inputs=++|
  Voltage Nuetral : Constant  Value=2.5
  Steering : Outport
  wires:
  Compass Heading/1 -> MATLAB Function/2(CompassHeading)
  Heading Desired/1 -> MATLAB Function/1(HeadingDesired)
  MATLAB Function/1(steering) -> Gain/1
  Gain/1 -> Sum/2
  Voltage Nuetral/1 -> Sum/1
  Sum/1 -> Saturation/1
  Saturation/1 -> Steering/1

== system RoboBoatVU_2014_Bacchus/Sinks/actuators/analog output/Subsystem/Propulsion Controller ==
  RPM : Inport
  Saturation : Saturate  UpperLimit=5  LowerLimit=0
  Sum : Sum  Inputs=++|
  Voltage Neutral : Constant  Value=2.5
  Volts / RPM : Gain  Gain=2.5/6000
  Propulsion : Outport
  wires:
  RPM/1 -> Volts / RPM/1
  Volts / RPM/1 -> Sum/2
  Voltage Neutral/1 -> Sum/1
  Sum/1 -> Saturation/1
  Saturation/1 -> Propulsion/1

== system RoboBoatVU_2014_Bacchus/Main FSM/Obstacle Navigation1/Obstacle Navigation/GPS: Bee Line/Approach/Output Heirarchy ==
  Nav Finished : Inport
  Desired Heading : Inport  Port=2
  Sensors : Inport  Port=3
  Annotated Image : Inport  Port=4
  Bus Creator : BusCreator  Inputs=3
  Bus Creator1 : BusCreator  Inputs=2
  Bus Creator2 : BusCreator  Inputs=3
  Bus Creator3 : BusCreator  Inputs=2
  Bus Creator4 : BusCreator  Inputs=2
  Due Sample Start : Constant  Value=0
  RPM Desired : Constant  Value=2000
  Ready to Read : Constant  Value=0
  Uno Power : Constant  Value=0
  Outputs : Outport
  wires:
  RPM Desired/1 -> Bus Creator/1  "RPM"
  Bus Creator/1 -> Bus Creator1/1  "Control Signals"
  Bus Creator2/1 -> Bus Creator/3  "Arduino Signals"
  Uno Power/1 -> Bus Creator2/2  "Uno Power"
  Desired Heading/1 -> Bus Creator/2  "Desired Heading"
  Bus Creator1/1 -> Bus Creator4/1  "Outputs"
  Annotated Image/1 -> Bus Creator1/2  "Annotated Image"
  Sensors/1 -> Bus Creator4/2  "Sensors"
  Bus Creator4/1 -> Bus Creator3/1  "Output Signals"
  Ready to Read/1 -> Bus Creator2/1  "Ready to Read"
  Due Sample Start/1 -> Bus Creator2/3  "Due Sample Start"
  Bus Creator3/1 -> Outputs/1
  Nav Finished/1 -> Bus Creator3/2  "Task Finished"

== system RoboBoatVU_2014_Bacchus/Main FSM/Obstacle Navigation1/Obstacle Navigation/GPS: Bee Line/Orient/Output Heirarchy1 ==
  Annotated Image : Inport
  Desired Heading : Inport  Port=2
  Sensors : Inport  Port=3
  Bus Creator : BusCreator  Inputs=3
  Bus Creator1 : BusCreator  Inputs=2
  Bus Creator2 : BusCreator  Inputs=3
  Bus Creator3 : BusCreator  Inputs=2
  Bus Creator4 : BusCreator  Inputs=2
  Due Sample Start : Constant  Value=0
  Finished : Constant  Value=0
  RPM Desired : Constant  Value=0
  Ready to Read : Constant  Value=0
  Uno Power : Constant  Value=0
  Outputs : Outport
  wires:
  RPM Desired/1 -> Bus Creator/1  "RPM"
  Bus Creator/1 -> Bus Creator1/1  "Control Signals"
  Bus Creator2/1 -> Bus Creator/3  "Arduino Signals"
  Uno Power/1 -> Bus Creator2/2  "Uno Power"
  Desired Heading/1 -> Bus Creator/2  "Desired Heading"
  Bus Creator1/1 -> Bus Creator4/1  "Outputs"
  Annotated Image/1 -> Bus Creator1/2  "Annotated Image"
  Sensors/1 -> Bus Creator4/2  "Sensors"
  Bus Creator4/1 -> Bus Creator3/1  "Output Signals"
  Ready to Read/1 -> Bus Creator2/1  "Ready to Read"
  Due Sample Start/1 -> Bus Creator2/3  "Due Sample Start"
  Bus Creator3/1 -> Outputs/1
  Finished/1 -> Bus Creator3/2  "Task Finished"
